simulink model "twistingTransferFunc"  (R2018b)
settings: Solver=VariableStepAuto  StartTime=0.0  StopTime=10.0  RelTol=1e-3  AbsTol=1e-3  EnableMultiTasking=on
settings Model: Creator=Mark Sherstan  LastModifiedBy=MarkSherstan
settings SolverCC: AutoScaleAbsTol=off
settings DataIOCC: LimitDataPoints=on  MaxDataPoints=10000
settings OptimizationCC: LifeSpan=inf
settings DebuggingCC: AllowSymbolicDim=off  LibraryContextMissingDiagnostic=none  SFUnexpectedBacktrackingDiag=warning  SFNoUnconditionalDefaultTransitionDiag=warning  SFExecutionAtInitializationDiag=none
settings SFSimCC: SimUseLocalCustomCode=off
settings RTWCC: RTWUseLocalCustomCode=off
settings CodeAppCC: StateflowObjectComments=on
settings GRTTargetCC: TargetLangStandard=C89/C90 (ANSI)  GeneratePreprocessorConditionals=Disable all
settings ConfigComp: CovMetricSettings=dw  CovHtmlReporting=on  CovSaveCumulativeToWorkspaceVar=on  CovSaveSingleToWorkspaceVar=on  CovExternalEMLEnable=off  CovSFcnEnable=off
settings SimscapeCC: SimscapeLogType=all  SimscapeLogDataHistory=10000

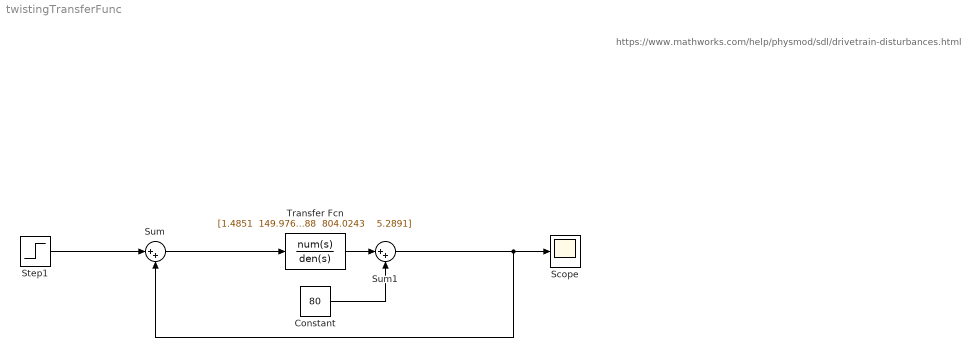
== system twistingTransferFunc ==
  note: https://www.mathworks.com/help/physmod/sdl/drivetrain-disturbances.html
  Constant : Constant  Value=80
  Scope : Scope
  Step1 : Step  Time=3  After=1000  SampleTime=0.0056
  Sum : Sum  Inputs=|++
  Sum1 : Sum  Inputs=|++
  Transfer Fcn : TransferFcn  Numerator="[1.4851  149.9761    2.3494]"  Denominator="[1.0000  108.9288  804.0243    5.2891]"
  wires:
  Step1/1 -> Sum/1
  Sum/1 -> Transfer Fcn/1
  Constant/1 -> Sum1/2
  Transfer Fcn/1 -> Sum1/1
  Sum1/1 -> Sum/2, Scope/1
